simulink model "Sim39"  (R2019a)
settings: Solver=FixedStepAuto  StartTime=0.0  StopTime=10.0  FixedStep=0.0001  RelTol=1e-3
settings Model: Creator=fbleo  LastModifiedBy=fbleo

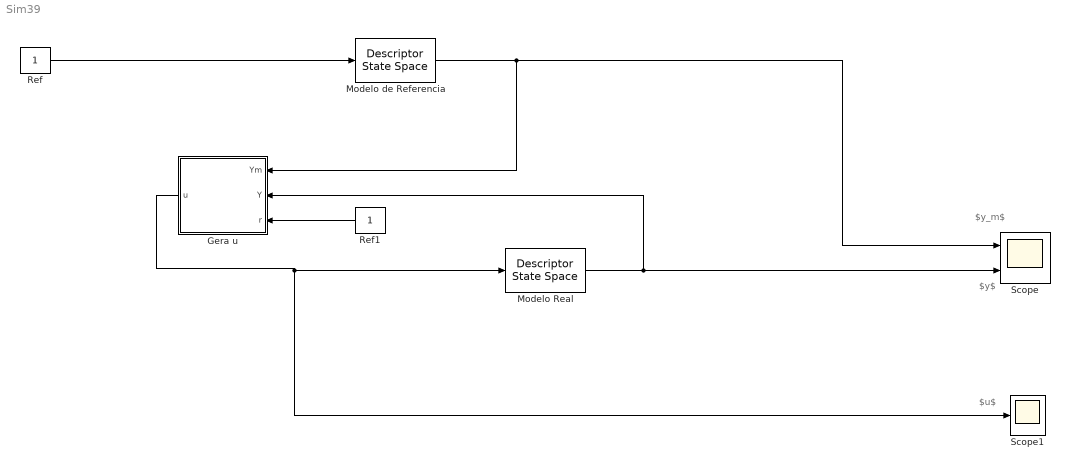
== system Sim39 ==
  note: $y$
  note: $u$
  note: $y_m$
  Gera u : Subsystem
  Modelo Real : DescriptorStateSpace  A=-1  B=2  D=0  InitialCondition=0.5
  Modelo de Referencia : DescriptorStateSpace  A=-3  B=3  D=0  InitialCondition=0
  Ref : Constant
  Ref1 : Constant
  Scope : Scope  NumInputPorts=2
  Scope1 : Scope
  wires:
  Modelo de Referencia/1 -> Scope/1, Gera u/1(Ym)
  Ref/1 -> Modelo de Referencia/1
  Gera u/1(u) -> Modelo Real/1, Scope1/1
  Modelo Real/1 -> Gera u/2(Y), Scope/2
  Ref1/1 -> Gera u/3(r)

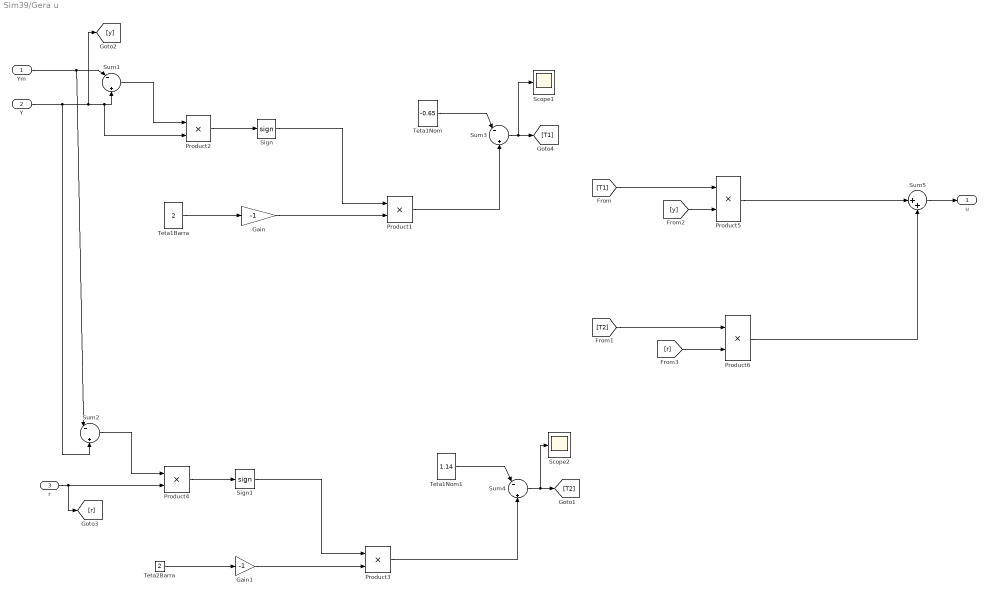
== system Sim39/Gera u ==
  Ym : Inport
  Y : Inport  Port=2
  r : Inport  Port=3
  Gain : Gain  Gain=-1
  Gain1 : Gain  Gain=-1
  Product{1..6} (6 alike) : Product
  Scope1 : Scope
  Scope2 : Scope
  Sign : Signum
  Sign1 : Signum
  Sum{1..4} (4 alike) : Sum  Inputs=|-||+
  Sum5 : Sum  Inputs=|++
  Teta1Barra : Constant  Value=2
  Teta1Nom : Constant  Value=-0.65
  Teta1Nom1 : Constant  Value=1.14
  Teta2Barra : Constant  Value=2
  u : Outport
  wires:
  Sign/1 -> Product1/1
  Gain/1 -> Product1/2
  Teta1Barra/1 -> Gain/1
  Sum1/1 -> Product2/1
  Product2/1 -> Sign/1
  Product1/1 -> Sum3/2
  Product3/1 -> Sum4/2
  Ym/1 -> Sum1/1, Sum2/1
  Sign1/1 -> Product3/1
  Product4/1 -> Sign1/1
  Sum2/1 -> Product4/1
  Gain1/1 -> Product3/2
  Y/1 -> [y], Product2/2, Sum1/2, Sum2/2
  Teta2Barra/1 -> Gain1/1
  r/1 -> [r], Product4/2
  [y] -> Product5/2
  [T2] -> Product6/1
  [r] -> Product6/2
  Product5/1 -> Sum5/1
  Product6/1 -> Sum5/2
  Sum5/1 -> u/1
  [T1] -> Product5/1
  Sum3/1 -> Scope1/1, [T1]
  Teta1Nom/1 -> Sum3/1
  Teta1Nom1/1 -> Sum4/1
  Sum4/1 -> Scope2/1, [T2]
